simulink model "Linear_Platform"  (R2022a)
settings: Solver=VariableStepAuto  StartTime=0.16733  StopTime=3000.0185  RelTol=1e-3
undefined symbols (not defined in the file): A_platform, B_platform, C_platform, L_platform
settings Model: Creator=ianam  LastModifiedBy=ianam
settings DataIOCC: InitialState=IC  LoadInitialState=on
settings DebuggingCC: UnderSpecifiedDataTypeMsg=error  UnderSpecifiedDimensionMsg=error

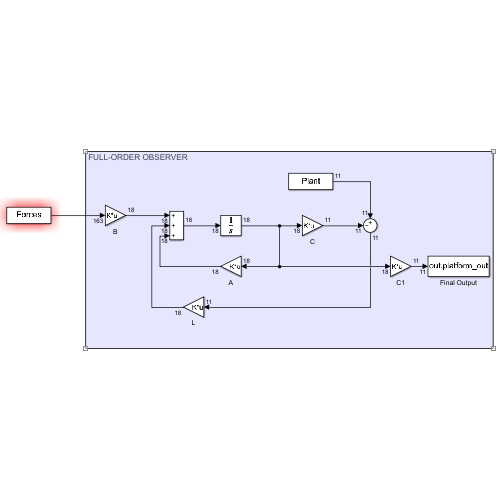
[thumbnail: Simulink's stored preview of the top-level diagram]
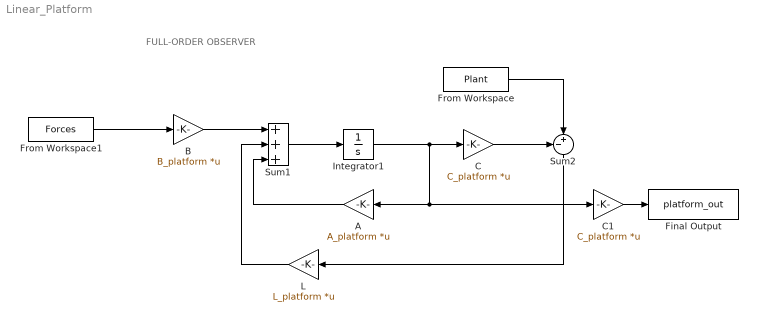
== system Linear_Platform ==
  note: FULL-ORDER OBSERVER
  A : Gain  Gain=A_platform  Multiplication=Matrix(K*u)
  B : Gain  Gain=B_platform  Multiplication=Matrix(K*u)
  C : Gain  Gain=C_platform  Multiplication=Matrix(K*u)
  C1 : Gain  Gain=C_platform  Multiplication=Matrix(K*u)
  Final Output : ToWorkspace  VariableName=platform_out  SaveFormat=Timeseries  SampleTime=-1
  From Workspace : FromWorkspace  VariableName=Plant
  From Workspace1 : FromWorkspace  VariableName=Forces
  Integrator1 : Integrator
  L : Gain  Gain=L_platform  Multiplication=Matrix(K*u)
  Sum1 : Sum  Inputs=+++
  Sum2 : Sum  Inputs=-+|
  wires:
  Sum1/1 -> Integrator1/1
  B/1 -> Sum1/1
  Integrator1/1 -> C1/1, A/1, C/1
  C/1 -> Sum2/1
  Sum2/1 -> L/1
  A/1 -> Sum1/3
  L/1 -> Sum1/2
  From Workspace/1 -> Sum2/2
  C1/1 -> Final Output/1
  From Workspace1/1 -> B/1
